simulink model "clik_inverse"  (Simulink 9.2)
settings: Solver=VariableStepAuto  StartTime=0.0  StopTime=4  RelTol=1e-3
values from neighbouring files (symbols this model uses):
  q0 = [-0.927293431585 -1.28700579042 0.7 2.21429922201]    [kinematic_traj.mat]
  Tc = 0.001    [kinematic_traj.mat]
undefined symbols (not defined in the file or in its folder): DiscIntNeverNeededParam
settings Model: Creator=josh7  LastModifiedBy=josh7  EnablePacing=on  PacingRate=0.890000
settings DataIOCC: LimitDataPoints=off  SaveFormat=Dataset  SignalLoggingSaveFormat=Dataset  ReturnWorkspaceOutputs=on
settings OptimizationCC: LifeSpan=auto
settings DebuggingCC: UnderspecifiedInitializationDetection=Simplified  MergeDetectMultiDrivingBlocksExec=error  FcnCallInpInsideContextMsg=error  StateNameClashWarn=none  SFUnexpectedBacktrackingDiag=error  SFNoUnconditionalDefaultTransitionDiag=error  SFExecutionAtInitializationDiag=warning
settings HardwareCC: ProdBitPerPointer=64  ProdBitPerSizeT=64  ProdBitPerPtrDiffT=64  ProdLargestAtomicFloat=Float  ProdIntDivRoundTo=Zero  ProdEndianess=LittleEndian  ProdWordSize=64  ProdHWDeviceType=Intel->x86-64 (Windows64)
settings ModelReferenceCC: PropagateSignalLabelsOutOfModel=on
settings SFSimCC: SimUseLocalCustomCode=on
settings RTWCC: RTWUseLocalCustomCode=on
settings CodeAppCC: StateflowObjectComments=off
settings GRTTargetCC: TargetLangStandard=C99 (ISO)  GeneratePreprocessorConditionals=Use local settings  CombineOutputUpdateFcns=on  GRTInterface=off
settings ConfigComp: CovMetricSettings=dwe  CovHtmlReporting=off  CovSaveCumulativeToWorkspaceVar=off  CovSaveSingleToWorkspaceVar=off  CovExternalEMLEnable=on

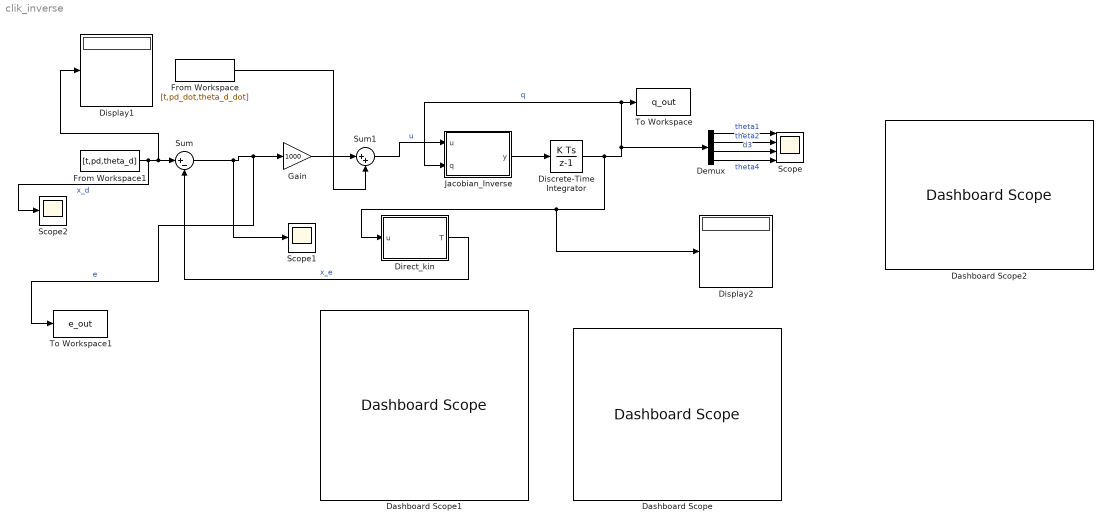
== system clik_inverse ==
  Dashboard Scope : DashboardScope
  Dashboard Scope1 : DashboardScope
  Dashboard Scope2 : DashboardScope
  Demux : Demux
  Direct_kin : MATLAB Function  TreatAsAtomicUnit=on
  Discrete-Time Integrator : DiscreteIntegrator  InitialCondition=q0  SampleTime=Tc  ICPrevOutput=DiscIntNeverNeededParam  ICPrevScaledInput=DiscIntNeverNeededParam
  Display1 : Display
  Display2 : Display
  From Workspace : FromWorkspace  VariableName=[t,pd_dot,theta_d_dot]  SampleTime=Tc
  From Workspace1 : FromWorkspace  VariableName=[t,pd,theta_d]  SampleTime=Tc
  Gain : Gain  Gain=1000
  Jacobian_Inverse : MATLAB Function  TreatAsAtomicUnit=on
  Scope : Scope  NumInputPorts=4
  Scope1 : Scope
  Scope2 : Scope
  Sum : Sum  Inputs=|+-
  Sum1 : Sum  Inputs=|++
  To Workspace : ToWorkspace  VariableName=q_out  SampleTime=-1
  To Workspace1 : ToWorkspace  VariableName=e_out  SampleTime=-1
  wires:
  Jacobian_Inverse/1(y) -> Discrete-Time Integrator/1
  Sum1/1 -> Jacobian_Inverse/1(u)  "u"
  Discrete-Time Integrator/1 -> Display2/1, Direct_kin/1(u), Demux/1, Jacobian_Inverse/2(q), To Workspace/1  "q"
  Gain/1 -> Sum1/1
  Direct_kin/1(T) -> Sum/2  "x_e"
  From Workspace/1 -> Sum1/2
  From Workspace1/1 -> Scope2/1, Display1/1, Sum/1  "x_d"
  Sum/1 -> Scope1/1, To Workspace1/1, Gain/1  "e"
  Demux/1 -> Scope/1  "theta1"
  Demux/2 -> Scope/2  "theta2"
  Demux/3 -> Scope/3  "d3"
  Demux/4 -> Scope/4  "theta4"

== matlab function Direct_kin ==
  data: u input double; T output double
function T = fcn(u)

a1=0.5;
a2 = 0.5;
b = u(1) + u(2);
c1 = cos(u(1));
s1 = sin(u(1));
c12 = cos(b);
s12 = sin(b);
d3=u(3);

T= [a2*c12+a1*c1;
    a2*s12+a1*s1;
    d3;
    u(1)+u(2)+u(4)];

== matlab function Jacobian_Inverse ==
  data: u input double; y output double; q input double
function y = fcn(u,q)

a1 = 0.5;
a2 = 0.5;
b = q(1)+q(2);
c1 = cos(q(1));
s1 = sin(q(1));
c12 = cos(b);
s12 = sin(b);


J = [-a2*s12-a1*s1 -a2*s12 0 0; 
    a2*c12+a1*c1 a2*c12 0 0; 
    0 0 1 0; 
    1 1 0 1];

y = inv(J)* u;
